simulink model "PID_controller"  (R2024a)
settings: Solver=FixedStepDiscrete  StartTime=0.0  StopTime=10  MaxStep=1e-3  RelTol=1e-3
undefined symbols (not defined in the file): DiscIntNeverNeededParam
libraries: simulink x2, pil_lib x1
settings Model: Creator=DELL  LastModifiedBy=DELL
settings OptimizationCC: DefaultParameterBehavior=Inlined  UseDivisionForNetSlopeComputation=on  GainParamInheritBuiltInType=on  UseFloatMulNetSlope=on  InlineInvariantSignals=on  PassReuseOutputArgsAs=Individual arguments  ZeroExternalMemoryAtStartup=off  ZeroInternalMemoryAtStartup=off  NoFixptDivByZeroProtection=on  EfficientFloat2IntCast=on  LifeSpan=1  OptimizeBlockOrder=speed  DifferentSizesBufferReuse=on  EfficientTunableParamExpr=on
settings DebuggingCC: ParameterTunabilityLossMsg=error
settings HardwareCC: ProdLongLongMode=on
settings SFSimCC: MATLABDynamicMemAlloc=off
settings RTWCC: Description=Embedded Coder  SystemTargetFile=ert.tlc  TemplateMakefile=ert_default_tmf  CreateSILPILBlock=SIL
settings CodeAppCC: ForceParamTrailComments=on  IgnoreCustomStorageClasses=off  OperatorAnnotations=on  SimulinkDataObjDesc=on  SFDataObjDesc=on  CustomSymbolStrGlobalVar=rt$N$M  CustomSymbolStrType=$N$M  CustomSymbolStrFcn=$N$M$F  CustomSymbolStrMacro=$N$M  InsertBlockDesc=on
settings ERTTargetCC: TargetLangStandard=C99 (ISO)  GenerateSampleERTMain=on  IncludeMdlTerminateFcn=off  CombineSignalStateStructs=on  SuppressErrorStatus=on  SupportAbsoluteTime=off  SupportComplex=off  InlinedParameterPlacement=NonHierarchical  ERTCustomFileTemplate=example_file_process.tlc  ERTFilePackagingFormat=CompactWithDataFile

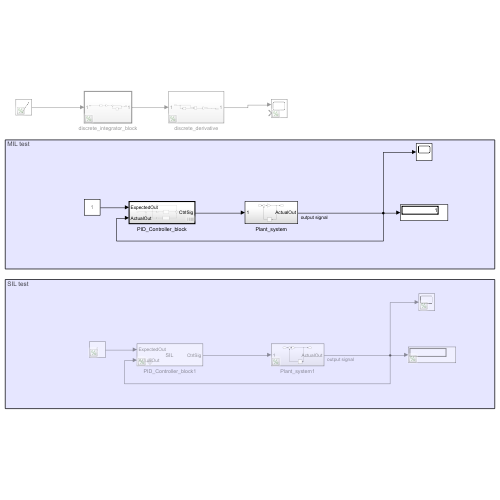
[thumbnail: Simulink's stored preview of the top-level diagram]
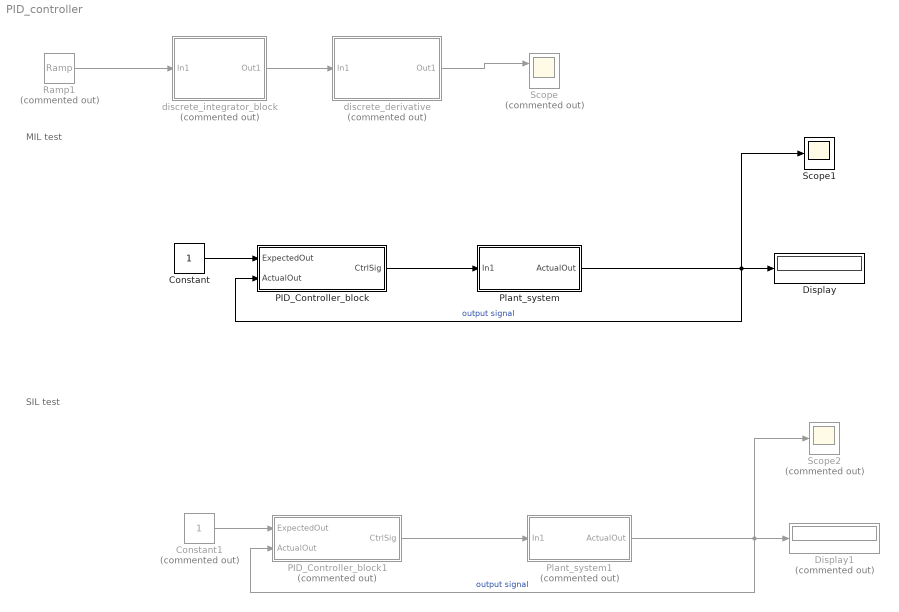
== system PID_controller ==
  note: SIL test
  note: MIL test
  Constant : Constant
  Constant1 : Constant  Commented=on
  Display : Display
  Display1 : Display  Commented=on
  PID_Controller_block : Subsystem  TreatAsAtomicUnit=on
  PID_Controller_block1 : Subsystem  Tag=__SL_testing_harness_stub_  Commented=on  DialogController=pil_create_dialog  LoadFcn=|
      | try
      |    if ~strcmp(rtw.pil.getPILVersion, '24.1 (R2024a)_15')
      |       set_param(gcb, 'DialogController', '');
      |       set_param(gcb, 'DialogControllerArgs', '');
      |    end
      | catch e
      |       set_param(gcb, 'DialogController', '');
      |       set_param(gcb, 'DialogControllerArgs', '');
      | end
      mask help: PIL:pil:XILBlockMaskDesc
      mask Display: disp('SIL');
  Plant_system : Subsystem
  Plant_system1 : Subsystem  Commented=on
  Ramp1 : simulink/Sources/Ramp  Commented=on  slope=1  start=0  InitialOutput=0
  Scope : Scope  Commented=on  NumInputPorts=2
  Scope1 : Scope
  Scope2 : Scope  Commented=on
  discrete_derivative : Subsystem  Commented=on
  discrete_integrator_block : Subsystem  Commented=on  TreatAsAtomicUnit=on
  wires:
  Constant/1 -> PID_Controller_block/1(ExpectedOut)
  Ramp1/1 -> discrete_integrator_block/1(In1)
  discrete_derivative/1(Out1) -> Scope/1
  discrete_integrator_block/1(Out1) -> discrete_derivative/1(In1)
  Constant1/1 -> PID_Controller_block1/1(ExpectedOut)
  Plant_system1/1(ActualOut) -> PID_Controller_block1/2(ActualOut), Display1/1, Scope2/1  "output signal"
  PID_Controller_block/1(CtrlSig) -> Plant_system/1(In1)
  Plant_system/1(ActualOut) -> PID_Controller_block/2(ActualOut), Display/1, Scope1/1  "output signal"
  PID_Controller_block1/1(CtrlSig) -> Plant_system1/1(In1)

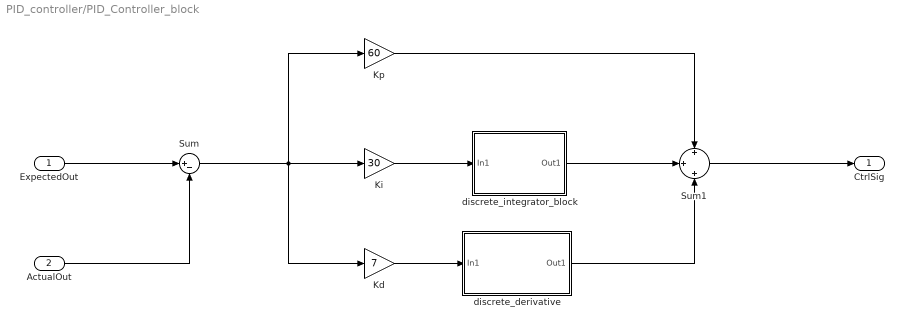
== system PID_controller/PID_Controller_block ==
  ExpectedOut : Inport
  ActualOut : Inport  Port=2
  Kd : Gain  Gain=7
  Ki : Gain  Gain=30
  Kp : Gain  Gain=60
  Sum : Sum  Inputs=|+-
  Sum1 : Sum  Inputs=+|+|+
  discrete_derivative : Subsystem  TreatAsAtomicUnit=on
  discrete_integrator_block : Subsystem  TreatAsAtomicUnit=on
  CtrlSig : Outport
  wires:
  discrete_derivative/1(Out1) -> Sum1/3
  Sum1/1 -> CtrlSig/1
  ActualOut/1 -> Sum/2
  discrete_integrator_block/1(Out1) -> Sum1/2
  ExpectedOut/1 -> Sum/1
  Sum/1 -> Ki/1, Kd/1, Kp/1
  Ki/1 -> discrete_integrator_block/1(In1)
  Kd/1 -> discrete_derivative/1(In1)
  Kp/1 -> Sum1/1

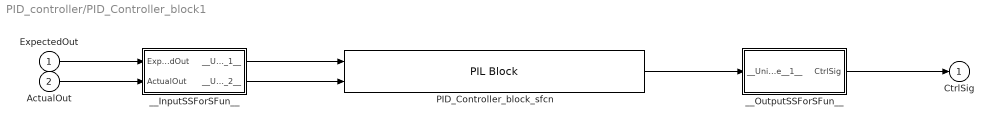
== system PID_controller/PID_Controller_block1 ==
  ExpectedOut : Inport
  ActualOut : Inport  Port=2
  PID_Controller_block_sfcn : pil_lib/PIL Block  SimulationMode=SIL  IsTopModelPIL=off  CodeDir=PID_Controller_block_ert_rtw  AnchorDir=C:\Users\DELL\Desktop\model-based-design\Section9_System_Modelling_Module\tasks\PID_MIL_SIL  ConfigName=Software-in-the-Loop (SIL)  XrelIsTopModelCode=on  XrelIsReusable=off  XrelDWorkNames={}  XrelDWorkTypes={}  XrelModelArgVals={}  XrelOrderedParamNames={}  XRelNonFiniteStyle=NONFINITE_UNUSED
  __InputSSForSFun__ : Subsystem
  __OutputSSForSFun__ : Subsystem
  CtrlSig : Outport
  wires:
  __OutputSSForSFun__/1(CtrlSig) -> CtrlSig/1
  PID_Controller_block_sfcn/1 -> __OutputSSForSFun__/1(__UniqueInportName__1__)
  __InputSSForSFun__/2(__UniqueOutportName__2__) -> PID_Controller_block_sfcn/2
  __InputSSForSFun__/1(__UniqueOutportName__1__) -> PID_Controller_block_sfcn/1
  ActualOut/1 -> __InputSSForSFun__/2(ActualOut)
  ExpectedOut/1 -> __InputSSForSFun__/1(ExpectedOut)

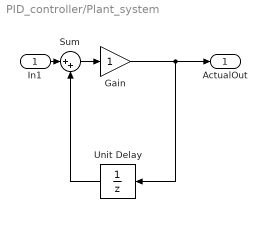
== system PID_controller/Plant_system ==
  In1 : Inport
  Gain : Gain
  Sum : Sum  Inputs=|++
  Unit Delay : UnitDelay  SampleTime=-1  HasFrameUpgradeWarning=on
  ActualOut : Outport
  wires:
  Gain/1 -> Unit Delay/1, ActualOut/1
  Unit Delay/1 -> Sum/2
  In1/1 -> Sum/1
  Sum/1 -> Gain/1

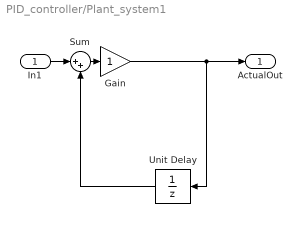
== system PID_controller/Plant_system1 ==
  In1 : Inport
  Gain : Gain
  Sum : Sum  Inputs=|++
  Unit Delay : UnitDelay  InitialCondition=1  SampleTime=-1  HasFrameUpgradeWarning=on
  ActualOut : Outport
  wires:
  Gain/1 -> Unit Delay/1, ActualOut/1
  Unit Delay/1 -> Sum/2
  Sum/1 -> Gain/1
  In1/1 -> Sum/1

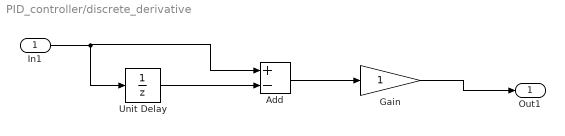
== system PID_controller/discrete_derivative ==
  In1 : Inport
  Add : Sum  Inputs=+-
  Gain : Gain
  Unit Delay : UnitDelay  SampleTime=-1  HasFrameUpgradeWarning=on
  Out1 : Outport
  wires:
  In1/1 -> Unit Delay/1, Add/1
  Gain/1 -> Out1/1
  Add/1 -> Gain/1
  Unit Delay/1 -> Add/2

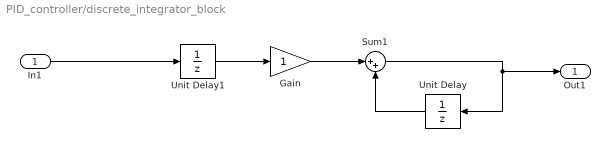
== system PID_controller/discrete_integrator_block ==
  In1 : Inport
  Gain : Gain
  Sum1 : Sum  Inputs=|++
  Unit Delay : UnitDelay  SampleTime=-1  HasFrameUpgradeWarning=on
  Unit Delay1 : UnitDelay  SampleTime=-1  HasFrameUpgradeWarning=on
  Out1 : Outport
  wires:
  In1/1 -> Unit Delay1/1
  Unit Delay/1 -> Sum1/2
  Sum1/1 -> Out1/1, Unit Delay/1
  Gain/1 -> Sum1/1
  Unit Delay1/1 -> Gain/1

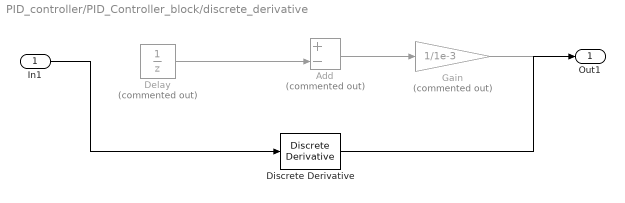
== system PID_controller/PID_Controller_block/discrete_derivative ==
  In1 : Inport
  Add : Sum  Commented=on  Inputs=+-
  Delay : UnitDelay  Commented=on  SampleTime=-1  HasFrameUpgradeWarning=on
  Discrete Derivative : simulink/Discrete/Discrete Derivative  gainval=1.0  ICPrevScaledInput=0.0  OutMin=[]  OutMax=[]  OutDataType=fixdt(1, 16)  OutScaling=2^-10  DoSatur=off
  Gain : Gain  Commented=on  Gain=1/1e-3
  Out1 : Outport
  wires:
  In1/1 -> Discrete Derivative/1
  Gain/1 -> ?
  Add/1 -> Gain/1
  Delay/1 -> Add/2
  Discrete Derivative/1 -> Out1/1

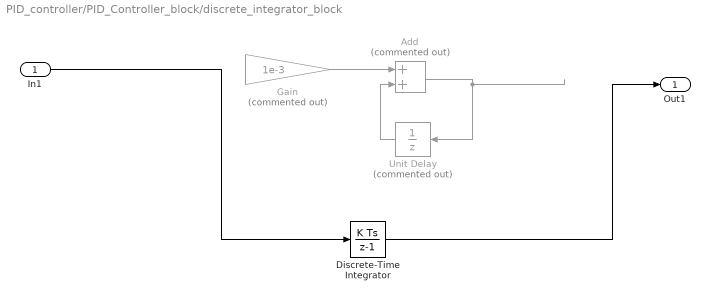
== system PID_controller/PID_Controller_block/discrete_integrator_block ==
  In1 : Inport
  Add : Sum  Commented=on
  Discrete-Time Integrator : DiscreteIntegrator  SampleTime=-1  ICPrevOutput=DiscIntNeverNeededParam  ICPrevScaledInput=DiscIntNeverNeededParam
  Gain : Gain  Commented=on  Gain=1e-3
  Unit Delay : UnitDelay  Commented=on  SampleTime=-1  HasFrameUpgradeWarning=on
  Out1 : Outport
  wires:
  Unit Delay/1 -> Add/2
  Add/1 -> Unit Delay/1
  Gain/1 -> Add/1
  In1/1 -> Discrete-Time Integrator/1
  Discrete-Time Integrator/1 -> Out1/1

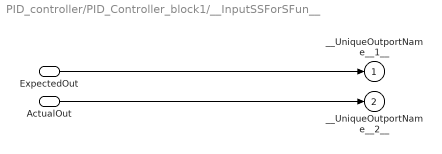
== system PID_controller/PID_Controller_block1/__InputSSForSFun__ ==
  ExpectedOut : Inport
  ActualOut : Inport  Port=2
  __UniqueOutportName__1__ : Outport
  __UniqueOutportName__2__ : Outport  Port=2
  wires:
  ActualOut/1 -> __UniqueOutportName__2__/1
  ExpectedOut/1 -> __UniqueOutportName__1__/1

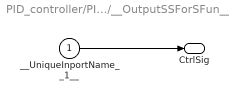
== system PID_controller/PID_Controller_block1/__OutputSSForSFun__ ==
  __UniqueInportName__1__ : Inport
  CtrlSig : Outport
  wires:
  __UniqueInportName__1__/1 -> CtrlSig/1
